simulink model "SF015A_WhlImbRejctn"  (R2013b)
settings: Solver=FixedStepDiscrete  SolverMode=SingleTasking  StartTime=0.0  StopTime=1  FixedStep=0.002  RelTol=1e-3
undefined symbols (not defined in the file): ACTIVBANDMAX_ULS_U32, ADAPVFILMAX_ULS_F32, ADJOUTPMAX_ULS_F32, ARCHGLBPRM_180OVERPI_ULS_F32, ARCHGLBPRM_2MILLISEC_SEC_F32, ARCHGLBPRM_2PI_ULS_F32, ARCHGLBPRM_FLOATZEROTHD_ULS_F32, ARCHGLBPRM_PI_ULS_F32, ARCHGLBPRM_PIOVER180_ULS_F32, ARCHGLBPRM_PIOVER2_ULS_F32, CALMINSPERCOUNT_ULS_F32, Cntr, DURATIONDISABLE_CNT_U16, FILTWHLSPDMAX_MOTRADPERSEC_F32, FRQMIN_ULS_F32, MICROSECTOMILLISEC_ULS_F32, MINSTOMILLISEC_ULS_F32, NINETY_ULS_F32, NODEBSTEP_CNT_U16, NROFDLY_CNT_U08, NtcSts1, NvmGetErrSts1, ONEHALF_ULS_F32, ONEHUNDRED_ULS_F32, ONEOVRTHREE_ULS_F32, ONEOVRTWENTY_ULS_F32, ONETHOUSAND_ULS_F32, PEAKMAX_ULS_F32, PEAKMIN_ULS_F32, PHAADJMAX_ULS_F32, PITIMESSAMPLETIME_ULS_F32, SigQlfr1, STOREDMINSPERCOUNT_ULS_F32, Sts, SysSt1, TWO_ULS_F32, TWOOVRTHREE_ULS_F32, UGRFILMAX_ULS_F32, WhlImbRejctnAdpvFac, WhlImbRejctnAutScaEna, WhlImbRejctnAutScaTar, WhlImbRejctnCurrMgnSlewPerLoop, WhlImbRejctnDcTrendFltRcvryDly, WhlImbRejctnDcTrendFltRcvryNegStep, WhlImbRejctnDcTrendFltRcvryPosStep, WhlImbRejctnDcTrendFltRcvryThd, WhlImbRejctnDcTrendTh2Tq, WhlImbRejctnDcTrendThTq, WhlImbRejctnDcTrendTi2Sec, WhlImbRejctnDcTrendTiSec, WhlImbRejctnEnaSlewPerLoop, WhlImbRejctnFctEna, WhlImbRejctnFltNtc, WhlImbRejctnFrqDiagcAmpThd, WhlImbRejctnFrqDiagcEna, WhlImbRejctnFrqDiagcFltRcvryDly, WhlImbRejctnFrqDiagcFltRcvryNegStep, WhlImbRejctnFrqDiagcFltRcvryPosStep, WhlImbRejctnFrqDiagcFltRcvryThd, WhlImbRejctnFrqDiagcThd ... (+30)
libraries: FixdToFloat x32, simulink x26, NxtrLim x25, Fil x20, NxtrAbslt x9, NxtrMath x7, NxtrMax x6, NxtrMin x4, NxtrNvM x2, FloatToFixd x2, LnrIntrpn x2, NxtrSign x1
(part 4 of 14)

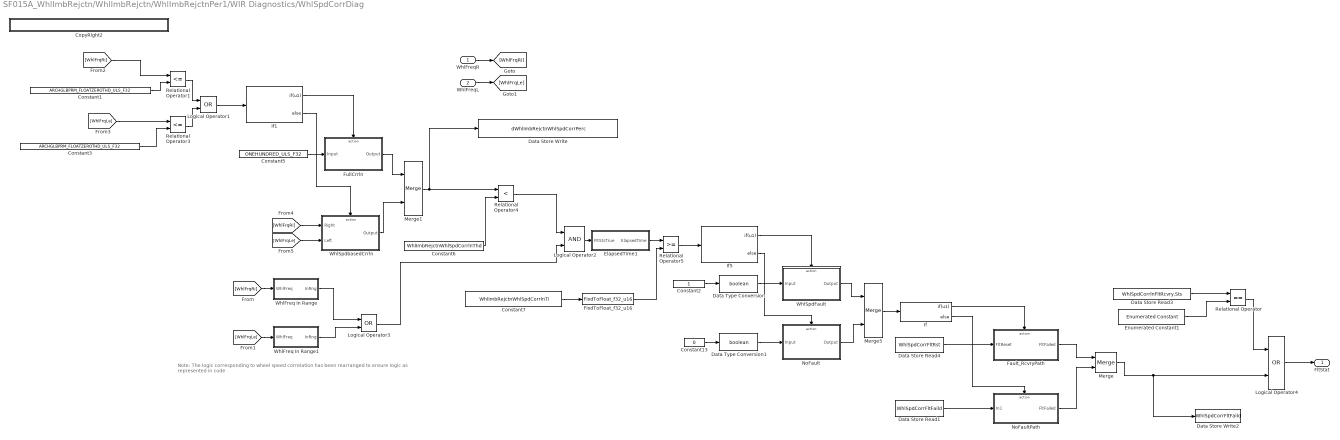
== system SF015A_WhlImbRejctn/WhlImbRejctn/WhlImbRejctnPer1/WIR Diagnostics/WhlSpdCorrDiag ==
  note: Note: The logic corresponding to wheel speed correlation has been rearranged to ensure logic as represented in code
  WhlFreqR : Inport
  WhlFreqL : Inport  Port=2
  Constant1 : Constant  Value=ARCHGLBPRM_FLOATZEROTHD_ULS_F32
  Constant13 : Constant  Value=0  OutDataTypeStr=boolean
  Constant2 : Constant  OutDataTypeStr=boolean
  Constant3 : Constant  Value=ARCHGLBPRM_FLOATZEROTHD_ULS_F32
  Constant5 : Constant  Value=ONEHUNDRED_ULS_F32
  Constant6 : Constant  Value=WhlImbRejctnWhlSpdCorrlnThd
  Constant7 : Constant  Value=WhlImbRejctnWhlSpdCorrlnTi
  CopyRight2 : Subsystem  Description=|  mask(Copyright Information){none=on}
      | Copyright info block.                                               
      |                                                                     
      | Place copyright information at the top of every subsystem in design.
      mask prompts: none "No parameters"
      mask help: Place copyright information at the top of every subsystem in design.
      mask Display:
      | NxtrConf = 'Nexteer Confidential';
      | 
      | sys = bdroot; %handle for the current model ("system")
      | first = get_param(sys,'Created');
      | first = first(end-3:end);  %year is last four digits
      | 
      | last = get_param(sys,'LastModifiedDate');
      | if isempty(last)
      |     last = datestr(now,'yyyy');
      | else
      |     last = last(end-3:end);
      | end
      | 
      | if strcmp(first,last)
      |     fprintf('%s -- Copyright %s Nexteer',NxtrConf,first)
      | else
      |     fprintf('%s -- %s%s- %s Nexteer',NxtrConf,char(169),first,last)
      | end
  Data Store Read1 : DataStoreRead  Priority=1  DataStoreName=WhlSpdCorrFltFaild
      settings: AttributesFormatString=Priority:%<Priority>
  Data Store Read3 : DataStoreRead  DataStoreName=WhlSpdCorrlnFltRcvry  DataStoreElements=WhlSpdCorrlnFltRcvry.Sts
  Data Store Read4 : DataStoreRead  Priority=1  DataStoreName=WhlSpdCorrFltRst
      settings: AttributesFormatString=Priority:%<Priority>
  Data Store Write : DataStoreWrite  DataStoreName=dWhlImbRejctnWhlSpdCorrPerc
  Data Store Write2 : DataStoreWrite  Priority=2  DataStoreName=WhlSpdCorrFltFaild
      settings: AttributesFormatString=Priority:%<Priority>
  Data Type Conversion : DataTypeConversion  OutDataTypeStr=boolean
  Data Type Conversion1 : DataTypeConversion  OutDataTypeStr=boolean
  ElapsedTime1 : Subsystem  TreatAsAtomicUnit=on
  Enumerated Constant1 : simulink/Sources/Enumerated Constant  OutDataTypeStr=Enum: SigQlfr1  Value=SigQlfr1.SIGQLFR_FAILD  SampleTime=inf
  Fault_RcvryPath : Subsystem  TreatAsAtomicUnit=on
  FixdToFloat_f32_u16 : FixdToFloat/FixdToFloat_f32_u16  Param1=0
  FullCrrln : Subsystem  RequirementInfo={} %GIDa_f316d04c_b5bf_4991_bd46_e1c3d0acec80  TreatAsAtomicUnit=on
  If : If  IfExpression=u1
  If1 : If  RequirementInfo={} %GIDa_4bc11ef0_d878_4cc4_82b4_0d0edb0129e4  IfExpression=u1
  If5 : If  RequirementInfo={} %GIDa_f8e2168d_295a_437f_93f0_d2de918d56ef  IfExpression=u1
  Logical Operator1 : Logic  Operator=OR  AllPortsSameDT=off  OutDataTypeStr=boolean
  Logical Operator2 : Logic  AllPortsSameDT=off  OutDataTypeStr=boolean
  Logical Operator3 : Logic  Operator=OR  AllPortsSameDT=off  OutDataTypeStr=boolean
  Logical Operator4 : Logic  Operator=OR  AllPortsSameDT=off  OutDataTypeStr=boolean
  Merge : Merge
  Merge1 : Merge
  Merge5 : Merge
  NoFault : Subsystem  RequirementInfo={} %GIDa_f7020847_ef3c_4257_9229_248ab4f76409  TreatAsAtomicUnit=on
  NoFaultPath : Subsystem  TreatAsAtomicUnit=on
  Relational Operator : RelationalOperator  Operator===  OutDataTypeStr=boolean
  Relational Operator1 : RelationalOperator  Operator=<=  OutDataTypeStr=boolean
  Relational Operator3 : RelationalOperator  Operator=<=  OutDataTypeStr=boolean
  Relational Operator4 : RelationalOperator  Operator=<  OutDataTypeStr=boolean
  Relational Operator5 : RelationalOperator  OutDataTypeStr=boolean
  WhlFreq In Range : Subsystem
  WhlFreq In Range1 : Subsystem
  WhlSpdFault : Subsystem  RequirementInfo={} %GIDa_32897d14_0a36_471e_bba2_f76c6f004030  TreatAsAtomicUnit=on
  WhlSpdbasedCrrln : Subsystem  RequirementInfo={} %GIDa_bfd7bd1e_da2d_43b7_9815_cea994d6f624  TreatAsAtomicUnit=on
  FltStat : Outport
  wires:
  Merge5/1 -> If/1
  Relational Operator1/1 -> Logical Operator1/1
  Relational Operator3/1 -> Logical Operator1/2
  Logical Operator1/1 -> If1/1
  Merge1/1 -> Data Store Write/1, Relational Operator4/1
  Constant6/1 -> Relational Operator4/2
  Constant7/1 -> FixdToFloat_f32_u16/1
  Relational Operator5/1 -> If5/1
  Relational Operator4/1 -> Logical Operator2/1
  WhlFreq In Range1/1(InRng) -> Logical Operator3/2
  WhlFreq In Range/1(InRng) -> Logical Operator3/1
  Logical Operator3/1 -> Logical Operator2/2
  If5/1 -> WhlSpdFault/Action
  If5/2 -> NoFault/Action
  WhlSpdFault/1(Output) -> Merge5/1
  NoFault/1(Output) -> Merge5/2
  Constant2/1 -> Data Type Conversion/1
  Constant13/1 -> Data Type Conversion1/1
  If1/1 -> FullCrrln/Action
  If1/2 -> WhlSpdbasedCrrln/Action
  FullCrrln/1(Output) -> Merge1/1
  WhlSpdbasedCrrln/1(Output) -> Merge1/2
  Constant5/1 -> FullCrrln/1(Input)
  ElapsedTime1/1(ElapsedTime) -> Relational Operator5/1
  Logical Operator2/1 -> ElapsedTime1/1(FltStsTrue)
  FixdToFloat_f32_u16/1 -> Relational Operator5/2
  Data Type Conversion/1 -> WhlSpdFault/1(Input)
  Data Type Conversion1/1 -> NoFault/1(Input)
  Constant3/1 -> Relational Operator3/2
  Constant1/1 -> Relational Operator1/2
  WhlFreqR/1 -> [WhlFrqRi]
  WhlFreqL/1 -> [WhlFrqLe]
  [WhlFrqRi] -> WhlFreq In Range/1(WhlFreq)
  [WhlFrqLe] -> WhlFreq In Range1/1(WhlFreq)
  [WhlFrqLe] -> Relational Operator3/1
  [WhlFrqRi] -> Relational Operator1/1
  [WhlFrqLe] -> WhlSpdbasedCrrln/2(Left)
  [WhlFrqRi] -> WhlSpdbasedCrrln/1(Right)
  Data Store Read4/1 -> Fault_RcvryPath/1(FltReset)
  If/1 -> Fault_RcvryPath/Action
  Fault_RcvryPath/1(FltFailed) -> Merge/1
  NoFaultPath/1(FltFailed) -> Merge/2
  If/2 -> NoFaultPath/Action
  Enumerated Constant1/1 -> Relational Operator/2
  Relational Operator/1 -> Logical Operator4/1
  Data Store Read3/1 -> Relational Operator/1
  Logical Operator4/1 -> FltStat/1
  Merge/1 -> Data Store Write2/1, Logical Operator4/2
  Data Store Read1/1 -> NoFaultPath/1(In1)

== system SF015A_WhlImbRejctn/WhlImbRejctn/WhlImbRejctnPer1/Whl Spd filter and Freq Estimation/CopyRight2 ==

== system SF015A_WhlImbRejctn/WhlImbRejctn/WhlImbRejctnPer1/Whl Spd filter and Freq Estimation/Tapped Delay ImplementationLe ==
  Input : Inport
  30 Delay's Execution : Subsystem  Priority=1  TreatAsAtomicUnit=on
      settings: AttributesFormatString=Priority:%<Priority>
  Assignment1 : Assignment  IndexMode=Zero-based  IndexOptions=Index vector (port)  Indices=1  OutputSizes=1
  Constant1 : Constant  Value=NROFDLY_CNT_U08  OutDataTypeStr=uint8
      settings: AttributesFormatString=%<OutDataTypeStr>
  CopyRight2 : Subsystem  Description=|  mask(Copyright Information){none=on}
      | Copyright info block.                                               
      |                                                                     
      | Place copyright information at the top of every subsystem in design.
      mask prompts: none "No parameters"
      mask help: Place copyright information at the top of every subsystem in design.
      mask Display:
      | NxtrConf = 'Nexteer Confidential';
      | 
      | sys = bdroot; %handle for the current model ("system")
      | first = get_param(sys,'Created');
      | first = first(end-3:end);  %year is last four digits
      | 
      | last = get_param(sys,'LastModifiedDate');
      | if isempty(last)
      |     last = datestr(now,'yyyy');
      | else
      |     last = last(end-3:end);
      | end
      | 
      | if strcmp(first,last)
      |     fprintf('%s -- Copyright %s Nexteer',NxtrConf,first)
      | else
      |     fprintf('%s -- %s%s- %s Nexteer',NxtrConf,char(169),first,last)
      | end
  Data Store Read1 : DataStoreRead  Priority=4  DataStoreName=StordValLe
      settings: AttributesFormatString=Priority=%<Priority>
  Data Store Read3 : DataStoreRead  Priority=2  DataStoreName=StordValLe
      settings: AttributesFormatString=Priority=%<Priority>
  Data Store Write : DataStoreWrite  Priority=3  DataStoreName=StordValLe
      settings: AttributesFormatString=Priority=%<Priority>
  Tapped Signal : Outport
  wires:
  Input/1 -> Assignment1/2
  Constant1/1 -> Assignment1/3
  Data Store Read3/1 -> Assignment1/1
  Assignment1/1 -> Data Store Write/1
  Data Store Read1/1 -> Tapped Signal/1

== system SF015A_WhlImbRejctn/WhlImbRejctn/WhlImbRejctnPer1/Whl Spd filter and Freq Estimation/Tapped Delay ImplementationRi ==
  Input : Inport
  30 Delay's Execution : Subsystem  Priority=1  TreatAsAtomicUnit=on
      settings: AttributesFormatString=Priority:%<Priority>
  Assignment1 : Assignment  IndexMode=Zero-based  IndexOptions=Index vector (port)  Indices=1  OutputSizes=1
  Constant1 : Constant  Value=NROFDLY_CNT_U08  OutDataTypeStr=uint8
      settings: AttributesFormatString=%<OutDataTypeStr>
  CopyRight2 : Subsystem  Description=|  mask(Copyright Information){none=on}
      | Copyright info block.                                               
      |                                                                     
      | Place copyright information at the top of every subsystem in design.
      mask prompts: none "No parameters"
      mask help: Place copyright information at the top of every subsystem in design.
      mask Display:
      | NxtrConf = 'Nexteer Confidential';
      | 
      | sys = bdroot; %handle for the current model ("system")
      | first = get_param(sys,'Created');
      | first = first(end-3:end);  %year is last four digits
      | 
      | last = get_param(sys,'LastModifiedDate');
      | if isempty(last)
      |     last = datestr(now,'yyyy');
      | else
      |     last = last(end-3:end);
      | end
      | 
      | if strcmp(first,last)
      |     fprintf('%s -- Copyright %s Nexteer',NxtrConf,first)
      | else
      |     fprintf('%s -- %s%s- %s Nexteer',NxtrConf,char(169),first,last)
      | end
  Data Store Read1 : DataStoreRead  Priority=4  DataStoreName=StordValRi
      settings: AttributesFormatString=Priority=%<Priority>
  Data Store Read3 : DataStoreRead  Priority=2  DataStoreName=StordValRi
      settings: AttributesFormatString=Priority=%<Priority>
  Data Store Write : DataStoreWrite  Priority=3  DataStoreName=StordValRi
      settings: AttributesFormatString=Priority=%<Priority>
  Tapped Signal : Outport
  wires:
  Input/1 -> Assignment1/2
  Constant1/1 -> Assignment1/3
  Data Store Read3/1 -> Assignment1/1
  Assignment1/1 -> Data Store Write/1
  Data Store Read1/1 -> Tapped Signal/1

== system SF015A_WhlImbRejctn/WhlImbRejctn/WhlImbRejctnPer1/Whl Spd filter and Freq Estimation/UGR L ==
  y : Inport
  FreqEst_Hz : Inport  Port=2
  PoleMag : Inport  Port=3
  Calc_ma1_a2 : Subsystem
  CopyRight2 : Subsystem  Description=|  mask(Copyright Information){none=on}
      | Copyright info block.                                               
      |                                                                     
      | Place copyright information at the top of every subsystem in design.
      mask prompts: none "No parameters"
      mask help: Place copyright information at the top of every subsystem in design.
      mask Display:
      | NxtrConf = 'Nexteer Confidential';
      | 
      | sys = bdroot; %handle for the current model ("system")
      | first = get_param(sys,'Created');
      | first = first(end-3:end);  %year is last four digits
      | 
      | last = get_param(sys,'LastModifiedDate');
      | if isempty(last)
      |     last = datestr(now,'yyyy');
      | else
      |     last = last(end-3:end);
      | end
      | 
      | if strcmp(first,last)
      |     fprintf('%s -- Copyright %s Nexteer',NxtrConf,first)
      | else
      |     fprintf('%s -- %s%s- %s Nexteer',NxtrConf,char(169),first,last)
      | end
  UnityGainResFilt : Subsystem
  y Filt : Outport
  wires:
  y/1 -> UnityGainResFilt/1(y)
  FreqEst_Hz/1 -> Calc_ma1_a2/1(f_est)
  UnityGainResFilt/1(Filt) -> y Filt/1
  Calc_ma1_a2/1(minus_a1) -> UnityGainResFilt/2(minus_a1)
  Calc_ma1_a2/2(a2) -> UnityGainResFilt/3(a2)
  PoleMag/1 -> Calc_ma1_a2/2(PoleMag)

== system SF015A_WhlImbRejctn/WhlImbRejctn/WhlImbRejctnPer1/Whl Spd filter and Freq Estimation/UGR R ==
  y : Inport
  FreqEst_Hz : Inport  Port=2
  PoleMag : Inport  Port=3
  Calc_ma1_a2 : Subsystem
  CopyRight2 : Subsystem  Description=|  mask(Copyright Information){none=on}
      | Copyright info block.                                               
      |                                                                     
      | Place copyright information at the top of every subsystem in design.
      mask prompts: none "No parameters"
      mask help: Place copyright information at the top of every subsystem in design.
      mask Display:
      | NxtrConf = 'Nexteer Confidential';
      | 
      | sys = bdroot; %handle for the current model ("system")
      | first = get_param(sys,'Created');
      | first = first(end-3:end);  %year is last four digits
      | 
      | last = get_param(sys,'LastModifiedDate');
      | if isempty(last)
      |     last = datestr(now,'yyyy');
      | else
      |     last = last(end-3:end);
      | end
      | 
      | if strcmp(first,last)
      |     fprintf('%s -- Copyright %s Nexteer',NxtrConf,first)
      | else
      |     fprintf('%s -- %s%s- %s Nexteer',NxtrConf,char(169),first,last)
      | end
  UnityGainResFilt : Subsystem
  y Filt : Outport
  wires:
  y/1 -> UnityGainResFilt/1(y)
  FreqEst_Hz/1 -> Calc_ma1_a2/1(f_est)
  UnityGainResFilt/1(Filt) -> y Filt/1
  Calc_ma1_a2/1(minus_a1) -> UnityGainResFilt/2(minus_a1)
  Calc_ma1_a2/2(a2) -> UnityGainResFilt/3(a2)
  PoleMag/1 -> Calc_ma1_a2/2(PoleMag)

== system SF015A_WhlImbRejctn/WhlImbRejctn/WhlImbRejctnPer2/Flt Recovery- DC Trend/CopyRight2 ==

== system SF015A_WhlImbRejctn/WhlImbRejctn/WhlImbRejctnPer2/Flt Recovery- DC Trend/ElapsedTime1 ==
  FltStsTrue : Inport
  CopyRight2 : Subsystem  Description=|  mask(Copyright Information){none=on}
      | Copyright info block.                                               
      |                                                                     
      | Place copyright information at the top of every subsystem in design.
      mask prompts: none "No parameters"
      mask help: Place copyright information at the top of every subsystem in design.
      mask Display:
      | NxtrConf = 'Nexteer Confidential';
      | 
      | sys = bdroot; %handle for the current model ("system")
      | first = get_param(sys,'Created');
      | first = first(end-3:end);  %year is last four digits
      | 
      | last = get_param(sys,'LastModifiedDate');
      | if isempty(last)
      |     last = datestr(now,'yyyy');
      | else
      |     last = last(end-3:end);
      | end
      | 
      | if strcmp(first,last)
      |     fprintf('%s -- Copyright %s Nexteer',NxtrConf,first)
      | else
      |     fprintf('%s -- %s%s- %s Nexteer',NxtrConf,char(169),first,last)
      | end
  Data Store Read : DataStoreRead  Priority=1  DataStoreName=DcTrendLrngEnaPrev
      settings: AttributesFormatString="priority:  %<Priority>"
  Data Store Write : DataStoreWrite  Priority=2  DataStoreName=DcTrendLrngEnaPrev
      settings: AttributesFormatString="priority:  %<Priority>"
  If : If  NumInputs=2  IfExpression=u1  ElseIfExpressions=u2
  If not true elapsed time = 0 : Subsystem  TreatAsAtomicUnit=on
  "If true and last step is true calculate elapsed time " : Subsystem  TreatAsAtomicUnit=on
  "If true and last step not true elapsed time = 0 get reference time " : Subsystem  TreatAsAtomicUnit=on
  Logical Operator1 : Logic  Operator=NOT  AllPortsSameDT=off  OutDataTypeStr=boolean
  Logical Operator2 : Logic  Operator=NOT  AllPortsSameDT=off  OutDataTypeStr=boolean
  Merge : Merge  Inputs=3
  ElapsedTime : Outport
  wires:
  If/1 -> If not true elapsed time = 0/Action
  If/2 -> "If true and last step not true elapsed time = 0 get reference time "/Action
  If/3 -> "If true and last step is true calculate elapsed time "/Action
  If not true elapsed time = 0/1(SpanTi) -> Merge/1
  "If true and last step not true elapsed time = 0 get reference time "/1("SpanTi ") -> Merge/2
  "If true and last step is true calculate elapsed time "/1(SpanTi) -> Merge/3
  Merge/1 -> ElapsedTime/1
  FltStsTrue/1 -> Logical Operator2/1, Data Store Write/1
  Data Store Read/1 -> Logical Operator1/1
  Logical Operator2/1 -> If/1
  Logical Operator1/1 -> If/2

== system SF015A_WhlImbRejctn/WhlImbRejctn/WhlImbRejctnPer2/Flt Recovery- DC Trend/FaultReset_Rcvry_False ==
  Action Port : ActionPort  ActionType=else
  Constant1 : Constant  Value=0  OutDataTypeStr=boolean
  CopyRight2 : Subsystem  Description=|  mask(Copyright Information){none=on}
      | Copyright info block.                                               
      |                                                                     
      | Place copyright information at the top of every subsystem in design.
      mask prompts: none "No parameters"
      mask help: Place copyright information at the top of every subsystem in design.
      mask Display:
      | NxtrConf = 'Nexteer Confidential';
      | 
      | sys = bdroot; %handle for the current model ("system")
      | first = get_param(sys,'Created');
      | first = first(end-3:end);  %year is last four digits
      | 
      | last = get_param(sys,'LastModifiedDate');
      | if isempty(last)
      |     last = datestr(now,'yyyy');
      | else
      |     last = last(end-3:end);
      | end
      | 
      | if strcmp(first,last)
      |     fprintf('%s -- Copyright %s Nexteer',NxtrConf,first)
      | else
      |     fprintf('%s -- %s%s- %s Nexteer',NxtrConf,char(169),first,last)
      | end
  Out1 : Outport
  wires:
  Constant1/1 -> Out1/1

== system SF015A_WhlImbRejctn/WhlImbRejctn/WhlImbRejctnPer2/Flt Recovery- DC Trend/FaultReset_Rcvry_True ==
  Action Port : ActionPort  ActionType=then
  Constant15 : Constant  OutDataTypeStr=boolean
  CopyRight2 : Subsystem  Description=|  mask(Copyright Information){none=on}
      | Copyright info block.                                               
      |                                                                     
      | Place copyright information at the top of every subsystem in design.
      mask prompts: none "No parameters"
      mask help: Place copyright information at the top of every subsystem in design.
      mask Display:
      | NxtrConf = 'Nexteer Confidential';
      | 
      | sys = bdroot; %handle for the current model ("system")
      | first = get_param(sys,'Created');
      | first = first(end-3:end);  %year is last four digits
      | 
      | last = get_param(sys,'LastModifiedDate');
      | if isempty(last)
      |     last = datestr(now,'yyyy');
      | else
      |     last = last(end-3:end);
      | end
      | 
      | if strcmp(first,last)
      |     fprintf('%s -- Copyright %s Nexteer',NxtrConf,first)
      | else
      |     fprintf('%s -- %s%s- %s Nexteer',NxtrConf,char(169),first,last)
      | end
  Out1 : Outport
  wires:
  Constant15/1 -> Out1/1

== system SF015A_WhlImbRejctn/WhlImbRejctn/WhlImbRejctnPer2/Flt Recovery- DC Trend/Update Fault Status ==
  Structvar : Inport
  Status : Inport  Port=2
  Bus Assignment : BusAssignment  AssignedSignals=Cntr,Sts
  Bus Selector : BusSelector  OutputSignals=Cntr,Sts,Thd,NegStep,PosStep
  Compare To Zero : simulink/Logic and Bit Operations/Compare To Zero  relop=<=  OutDataTypeStr=boolean
  Constant : Constant  Value=0  OutDataTypeStr=single
  CopyRight2 : Subsystem  Description=|  mask(Copyright Information){none=on}
      | Copyright info block.                                               
      |                                                                     
      | Place copyright information at the top of every subsystem in design.
      mask prompts: none "No parameters"
      mask help: Place copyright information at the top of every subsystem in design.
      mask Display:
      | NxtrConf = 'Nexteer Confidential';
      | 
      | sys = bdroot; %handle for the current model ("system")
      | first = get_param(sys,'Created');
      | first = first(end-3:end);  %year is last four digits
      | 
      | last = get_param(sys,'LastModifiedDate');
      | if isempty(last)
      |     last = datestr(now,'yyyy');
      | else
      |     last = last(end-3:end);
      | end
      | 
      | if strcmp(first,last)
      |     fprintf('%s -- Copyright %s Nexteer',NxtrConf,first)
      | else
      |     fprintf('%s -- %s%s- %s Nexteer',NxtrConf,char(169),first,last)
      | end
  Enumerated Constant : simulink/Sources/Enumerated Constant  OutDataTypeStr=Enum: SigQlfr1  Value=SigQlfr1.SIGQLFR_FAILD  SampleTime=inf
  Enumerated Constant1 : simulink/Sources/Enumerated Constant  OutDataTypeStr=Enum: SigQlfr1  Value=SigQlfr1.SIGQLFR_PASSD  SampleTime=inf
  If : If  IfExpression=u1
  If1 : If  NumInputs=2  IfExpression=u1  ElseIfExpressions=u2  ShowElse=off
  Merge : Merge
  Relational Operator : RelationalOperator  OutDataTypeStr=boolean
  Terminator : Terminator
  Towards Failed : Subsystem  TreatAsAtomicUnit=on
  Towards Passed : Subsystem  TreatAsAtomicUnit=on
  Update to Failed : Subsystem  TreatAsAtomicUnit=on
  Update to Passed : Subsystem  TreatAsAtomicUnit=on
  counter : Merge
  Structvar_out : Outport
  wires:
  Structvar/1 -> Bus Assignment/1, Bus Selector/1
  Status/1 -> If/1
  If/1 -> Towards Failed/Action
  If/2 -> Towards Passed/Action
  [PosStep] -> Towards Failed/1(PosStep)
  [NegStep] -> Towards Passed/1(NegStep)
  Towards Failed/1(Out1) -> counter/1
  Towards Passed/1(Out1) -> counter/2
  [Cnt] -> Towards Failed/2(Cnt)
  [Thd] -> Towards Failed/3(Thd)
  Constant/1 -> Towards Passed/3(Thd)
  counter/1 -> [Cnt_update], Compare To Zero/1, Relational Operator/1
  Relational Operator/1 -> If1/1
  If1/1 -> Update to Failed/Action
  If1/2 -> Update to Passed/Action
  Compare To Zero/1 -> If1/2
  Enumerated Constant1/1 -> Update to Passed/1(In1)
  Update to Failed/1(Out1) -> Merge/1
  Update to Passed/1(Out1) -> Merge/2
  Enumerated Constant/1 -> Update to Failed/1(In1)
  Bus Assignment/1 -> Structvar_out/1
  Merge/1 -> [Sts_update]
  Bus Selector/1 -> [Cnt]  "<Cntr>"
  Bus Selector/3 -> [Thd]  "<Thd>"
  Bus Selector/4 -> [NegStep]  "<NegStep>"
  Bus Selector/5 -> [PosStep]  "<PosStep>"
  [Cnt_update] -> Bus Assignment/2
  [Sts_update] -> Bus Assignment/3
  [Cnt] -> Towards Passed/2(Cnt)
  [Thd] -> Relational Operator/2
  Bus Selector/2 -> Terminator/1  "<Sts>"

== system SF015A_WhlImbRejctn/WhlImbRejctn/WhlImbRejctnPer2/Flt Recovery- Freq Diag/CopyRight2 ==

== system SF015A_WhlImbRejctn/WhlImbRejctn/WhlImbRejctnPer2/Flt Recovery- Freq Diag/ElapsedTime1 ==
  FltStsTrue : Inport
  CopyRight2 : Subsystem  Description=|  mask(Copyright Information){none=on}
      | Copyright info block.                                               
      |                                                                     
      | Place copyright information at the top of every subsystem in design.
      mask prompts: none "No parameters"
      mask help: Place copyright information at the top of every subsystem in design.
      mask Display:
      | NxtrConf = 'Nexteer Confidential';
      | 
      | sys = bdroot; %handle for the current model ("system")
      | first = get_param(sys,'Created');
      | first = first(end-3:end);  %year is last four digits
      | 
      | last = get_param(sys,'LastModifiedDate');
      | if isempty(last)
      |     last = datestr(now,'yyyy');
      | else
      |     last = last(end-3:end);
      | end
      | 
      | if strcmp(first,last)
      |     fprintf('%s -- Copyright %s Nexteer',NxtrConf,first)
      | else
      |     fprintf('%s -- %s%s- %s Nexteer',NxtrConf,char(169),first,last)
      | end
  Data Store Read : DataStoreRead  Priority=1  DataStoreName=FrqDiagcLrngEnaPrev
      settings: AttributesFormatString="priority:  %<Priority>"
  Data Store Write : DataStoreWrite  Priority=2  DataStoreName=FrqDiagcLrngEnaPrev
      settings: AttributesFormatString="priority:  %<Priority>"
  If : If  NumInputs=2  IfExpression=u1  ElseIfExpressions=u2
  If not true elapsed time = 0 : Subsystem  TreatAsAtomicUnit=on
  "If true and last step is true calculate elapsed time " : Subsystem  TreatAsAtomicUnit=on
  "If true and last step not true elapsed time = 0 get reference time " : Subsystem  TreatAsAtomicUnit=on
  Logical Operator1 : Logic  Operator=NOT  AllPortsSameDT=off  OutDataTypeStr=boolean
  Logical Operator2 : Logic  Operator=NOT  AllPortsSameDT=off  OutDataTypeStr=boolean
  Merge : Merge  Inputs=3
  ElapsedTime : Outport
  wires:
  If/1 -> If not true elapsed time = 0/Action
  If/2 -> "If true and last step not true elapsed time = 0 get reference time "/Action
  If/3 -> "If true and last step is true calculate elapsed time "/Action
  If not true elapsed time = 0/1(SpanTi) -> Merge/1
  "If true and last step not true elapsed time = 0 get reference time "/1("SpanTi ") -> Merge/2
  "If true and last step is true calculate elapsed time "/1(SpanTi) -> Merge/3
  Merge/1 -> ElapsedTime/1
  FltStsTrue/1 -> Logical Operator2/1, Data Store Write/1
  Data Store Read/1 -> Logical Operator1/1
  Logical Operator2/1 -> If/1
  Logical Operator1/1 -> If/2

== system SF015A_WhlImbRejctn/WhlImbRejctn/WhlImbRejctnPer2/Flt Recovery- Freq Diag/FaultReset_Rcvry_False ==
  Action Port : ActionPort  ActionType=else
  Constant1 : Constant  Value=0  OutDataTypeStr=boolean
  CopyRight2 : Subsystem  Description=|  mask(Copyright Information){none=on}
      | Copyright info block.                                               
      |                                                                     
      | Place copyright information at the top of every subsystem in design.
      mask prompts: none "No parameters"
      mask help: Place copyright information at the top of every subsystem in design.
      mask Display:
      | NxtrConf = 'Nexteer Confidential';
      | 
      | sys = bdroot; %handle for the current model ("system")
      | first = get_param(sys,'Created');
      | first = first(end-3:end);  %year is last four digits
      | 
      | last = get_param(sys,'LastModifiedDate');
      | if isempty(last)
      |     last = datestr(now,'yyyy');
      | else
      |     last = last(end-3:end);
      | end
      | 
      | if strcmp(first,last)
      |     fprintf('%s -- Copyright %s Nexteer',NxtrConf,first)
      | else
      |     fprintf('%s -- %s%s- %s Nexteer',NxtrConf,char(169),first,last)
      | end
  Out1 : Outport
  wires:
  Constant1/1 -> Out1/1

== system SF015A_WhlImbRejctn/WhlImbRejctn/WhlImbRejctnPer2/Flt Recovery- Freq Diag/FaultReset_Rcvry_True ==
  Action Port : ActionPort  ActionType=then
  Constant15 : Constant  OutDataTypeStr=boolean
  CopyRight2 : Subsystem  Description=|  mask(Copyright Information){none=on}
      | Copyright info block.                                               
      |                                                                     
      | Place copyright information at the top of every subsystem in design.
      mask prompts: none "No parameters"
      mask help: Place copyright information at the top of every subsystem in design.
      mask Display:
      | NxtrConf = 'Nexteer Confidential';
      | 
      | sys = bdroot; %handle for the current model ("system")
      | first = get_param(sys,'Created');
      | first = first(end-3:end);  %year is last four digits
      | 
      | last = get_param(sys,'LastModifiedDate');
      | if isempty(last)
      |     last = datestr(now,'yyyy');
      | else
      |     last = last(end-3:end);
      | end
      | 
      | if strcmp(first,last)
      |     fprintf('%s -- Copyright %s Nexteer',NxtrConf,first)
      | else
      |     fprintf('%s -- %s%s- %s Nexteer',NxtrConf,char(169),first,last)
      | end
  Out1 : Outport
  wires:
  Constant15/1 -> Out1/1

== system SF015A_WhlImbRejctn/WhlImbRejctn/WhlImbRejctnPer2/Flt Recovery- Freq Diag/Update Fault Status ==
  Structvar : Inport
  Status : Inport  Port=2
  Bus Assignment : BusAssignment  AssignedSignals=Cntr,Sts
  Bus Selector : BusSelector  OutputSignals=Cntr,Sts,Thd,NegStep,PosStep
  Compare To Zero : simulink/Logic and Bit Operations/Compare To Zero  relop=<=  OutDataTypeStr=boolean
  Constant : Constant  Value=0  OutDataTypeStr=single
  CopyRight2 : Subsystem  Description=|  mask(Copyright Information){none=on}
      | Copyright info block.                                               
      |                                                                     
      | Place copyright information at the top of every subsystem in design.
      mask prompts: none "No parameters"
      mask help: Place copyright information at the top of every subsystem in design.
      mask Display:
      | NxtrConf = 'Nexteer Confidential';
      | 
      | sys = bdroot; %handle for the current model ("system")
      | first = get_param(sys,'Created');
      | first = first(end-3:end);  %year is last four digits
      | 
      | last = get_param(sys,'LastModifiedDate');
      | if isempty(last)
      |     last = datestr(now,'yyyy');
      | else
      |     last = last(end-3:end);
      | end
      | 
      | if strcmp(first,last)
      |     fprintf('%s -- Copyright %s Nexteer',NxtrConf,first)
      | else
      |     fprintf('%s -- %s%s- %s Nexteer',NxtrConf,char(169),first,last)
      | end
  Enumerated Constant : simulink/Sources/Enumerated Constant  OutDataTypeStr=Enum: SigQlfr1  Value=SigQlfr1.SIGQLFR_FAILD  SampleTime=inf
  Enumerated Constant1 : simulink/Sources/Enumerated Constant  OutDataTypeStr=Enum: SigQlfr1  Value=SigQlfr1.SIGQLFR_PASSD  SampleTime=inf
  If : If  IfExpression=u1
  If1 : If  NumInputs=2  IfExpression=u1  ElseIfExpressions=u2  ShowElse=off
  Merge : Merge
  Relational Operator : RelationalOperator  OutDataTypeStr=boolean
  Terminator : Terminator
  Towards Failed : Subsystem  TreatAsAtomicUnit=on
  Towards Passed : Subsystem  TreatAsAtomicUnit=on
  Update to Failed : Subsystem  TreatAsAtomicUnit=on
  Update to Passed : Subsystem  TreatAsAtomicUnit=on
  counter : Merge
  Structvar_out : Outport
  wires:
  Structvar/1 -> Bus Assignment/1, Bus Selector/1
  Status/1 -> If/1
  If/1 -> Towards Failed/Action
  If/2 -> Towards Passed/Action
  [PosStep] -> Towards Failed/1(PosStep)
  [NegStep] -> Towards Passed/1(NegStep)
  Towards Failed/1(Out1) -> counter/1
  Towards Passed/1(Out1) -> counter/2
  [Cnt] -> Towards Failed/2(Cnt)
  [Thd] -> Towards Failed/3(Thd)
  Constant/1 -> Towards Passed/3(Thd)
  counter/1 -> [Cnt_update], Compare To Zero/1, Relational Operator/1
  Relational Operator/1 -> If1/1
  If1/1 -> Update to Failed/Action
  If1/2 -> Update to Passed/Action
  Compare To Zero/1 -> If1/2
  Enumerated Constant1/1 -> Update to Passed/1(In1)
  Update to Failed/1(Out1) -> Merge/1
  Update to Passed/1(Out1) -> Merge/2
  Enumerated Constant/1 -> Update to Failed/1(In1)
  Bus Assignment/1 -> Structvar_out/1
  Merge/1 -> [Sts_update]
  Bus Selector/1 -> [Cnt]  "<Cntr>"
  Bus Selector/3 -> [Thd]  "<Thd>"
  Bus Selector/4 -> [NegStep]  "<NegStep>"
  Bus Selector/5 -> [PosStep]  "<PosStep>"
  [Cnt_update] -> Bus Assignment/2
  [Sts_update] -> Bus Assignment/3
  [Cnt] -> Towards Passed/2(Cnt)
  [Thd] -> Relational Operator/2
  Bus Selector/2 -> Terminator/1  "<Sts>"

== system SF015A_WhlImbRejctn/WhlImbRejctn/WhlImbRejctnPer2/Flt Recovery- Max Mag/CopyRight2 ==

== system SF015A_WhlImbRejctn/WhlImbRejctn/WhlImbRejctnPer2/Flt Recovery- Max Mag/ElapsedTime1 ==
  FltStsTrue : Inport
  CopyRight2 : Subsystem  Description=|  mask(Copyright Information){none=on}
      | Copyright info block.                                               
      |                                                                     
      | Place copyright information at the top of every subsystem in design.
      mask prompts: none "No parameters"
      mask help: Place copyright information at the top of every subsystem in design.
      mask Display:
      | NxtrConf = 'Nexteer Confidential';
      | 
      | sys = bdroot; %handle for the current model ("system")
      | first = get_param(sys,'Created');
      | first = first(end-3:end);  %year is last four digits
      | 
      | last = get_param(sys,'LastModifiedDate');
      | if isempty(last)
      |     last = datestr(now,'yyyy');
      | else
      |     last = last(end-3:end);
      | end
      | 
      | if strcmp(first,last)
      |     fprintf('%s -- Copyright %s Nexteer',NxtrConf,first)
      | else
      |     fprintf('%s -- %s%s- %s Nexteer',NxtrConf,char(169),first,last)
      | end
  Data Store Read : DataStoreRead  Priority=1  DataStoreName=MaxMgnLrngEnaPrev
      settings: AttributesFormatString="priority:  %<Priority>"
  Data Store Write : DataStoreWrite  Priority=2  DataStoreName=MaxMgnLrngEnaPrev
      settings: AttributesFormatString="priority:  %<Priority>"
  If : If  NumInputs=2  IfExpression=u1  ElseIfExpressions=u2
  If not true elapsed time = 0 : Subsystem  TreatAsAtomicUnit=on
  "If true and last step is true calculate elapsed time " : Subsystem  TreatAsAtomicUnit=on
  "If true and last step not true elapsed time = 0 get reference time " : Subsystem  TreatAsAtomicUnit=on
  Logical Operator1 : Logic  Operator=NOT  AllPortsSameDT=off  OutDataTypeStr=boolean
  Logical Operator2 : Logic  Operator=NOT  AllPortsSameDT=off  OutDataTypeStr=boolean
  Merge : Merge  Inputs=3
  ElapsedTime : Outport
  wires:
  If/1 -> If not true elapsed time = 0/Action
  If/2 -> "If true and last step not true elapsed time = 0 get reference time "/Action
  If/3 -> "If true and last step is true calculate elapsed time "/Action
  If not true elapsed time = 0/1(SpanTi) -> Merge/1
  "If true and last step not true elapsed time = 0 get reference time "/1("SpanTi ") -> Merge/2
  "If true and last step is true calculate elapsed time "/1(SpanTi) -> Merge/3
  Merge/1 -> ElapsedTime/1
  FltStsTrue/1 -> Logical Operator2/1, Data Store Write/1
  Data Store Read/1 -> Logical Operator1/1
  Logical Operator2/1 -> If/1
  Logical Operator1/1 -> If/2

== system SF015A_WhlImbRejctn/WhlImbRejctn/WhlImbRejctnPer2/Flt Recovery- Max Mag/FaultReset_Rcvry_False ==
  Action Port : ActionPort  ActionType=else
  Constant1 : Constant  Value=0  OutDataTypeStr=boolean
  CopyRight2 : Subsystem  Description=|  mask(Copyright Information){none=on}
      | Copyright info block.                                               
      |                                                                     
      | Place copyright information at the top of every subsystem in design.
      mask prompts: none "No parameters"
      mask help: Place copyright information at the top of every subsystem in design.
      mask Display:
      | NxtrConf = 'Nexteer Confidential';
      | 
      | sys = bdroot; %handle for the current model ("system")
      | first = get_param(sys,'Created');
      | first = first(end-3:end);  %year is last four digits
      | 
      | last = get_param(sys,'LastModifiedDate');
      | if isempty(last)
      |     last = datestr(now,'yyyy');
      | else
      |     last = last(end-3:end);
      | end
      | 
      | if strcmp(first,last)
      |     fprintf('%s -- Copyright %s Nexteer',NxtrConf,first)
      | else
      |     fprintf('%s -- %s%s- %s Nexteer',NxtrConf,char(169),first,last)
      | end
  Out1 : Outport
  wires:
  Constant1/1 -> Out1/1

== system SF015A_WhlImbRejctn/WhlImbRejctn/WhlImbRejctnPer2/Flt Recovery- Max Mag/FaultReset_Rcvry_True ==
  Action Port : ActionPort  ActionType=then
  Constant15 : Constant  OutDataTypeStr=boolean
  CopyRight2 : Subsystem  Description=|  mask(Copyright Information){none=on}
      | Copyright info block.                                               
      |                                                                     
      | Place copyright information at the top of every subsystem in design.
      mask prompts: none "No parameters"
      mask help: Place copyright information at the top of every subsystem in design.
      mask Display:
      | NxtrConf = 'Nexteer Confidential';
      | 
      | sys = bdroot; %handle for the current model ("system")
      | first = get_param(sys,'Created');
      | first = first(end-3:end);  %year is last four digits
      | 
      | last = get_param(sys,'LastModifiedDate');
      | if isempty(last)
      |     last = datestr(now,'yyyy');
      | else
      |     last = last(end-3:end);
      | end
      | 
      | if strcmp(first,last)
      |     fprintf('%s -- Copyright %s Nexteer',NxtrConf,first)
      | else
      |     fprintf('%s -- %s%s- %s Nexteer',NxtrConf,char(169),first,last)
      | end
  Out1 : Outport
  wires:
  Constant15/1 -> Out1/1

== system SF015A_WhlImbRejctn/WhlImbRejctn/WhlImbRejctnPer2/Flt Recovery- Max Mag/Update Fault Status ==
  Structvar : Inport
  Status : Inport  Port=2
  Bus Assignment : BusAssignment  AssignedSignals=Cntr,Sts
  Bus Selector : BusSelector  OutputSignals=Cntr,Sts,Thd,NegStep,PosStep
  Compare To Zero : simulink/Logic and Bit Operations/Compare To Zero  relop=<=  OutDataTypeStr=boolean
  Constant : Constant  Value=0  OutDataTypeStr=single
  CopyRight2 : Subsystem  Description=|  mask(Copyright Information){none=on}
      | Copyright info block.                                               
      |                                                                     
      | Place copyright information at the top of every subsystem in design.
      mask prompts: none "No parameters"
      mask help: Place copyright information at the top of every subsystem in design.
      mask Display:
      | NxtrConf = 'Nexteer Confidential';
      | 
      | sys = bdroot; %handle for the current model ("system")
      | first = get_param(sys,'Created');
      | first = first(end-3:end);  %year is last four digits
      | 
      | last = get_param(sys,'LastModifiedDate');
      | if isempty(last)
      |     last = datestr(now,'yyyy');
      | else
      |     last = last(end-3:end);
      | end
      | 
      | if strcmp(first,last)
      |     fprintf('%s -- Copyright %s Nexteer',NxtrConf,first)
      | else
      |     fprintf('%s -- %s%s- %s Nexteer',NxtrConf,char(169),first,last)
      | end
  Enumerated Constant : simulink/Sources/Enumerated Constant  OutDataTypeStr=Enum: SigQlfr1  Value=SigQlfr1.SIGQLFR_FAILD  SampleTime=inf
  Enumerated Constant1 : simulink/Sources/Enumerated Constant  OutDataTypeStr=Enum: SigQlfr1  Value=SigQlfr1.SIGQLFR_PASSD  SampleTime=inf
  If : If  IfExpression=u1
  If1 : If  NumInputs=2  IfExpression=u1  ElseIfExpressions=u2  ShowElse=off
  Merge : Merge
  Relational Operator : RelationalOperator  OutDataTypeStr=boolean
  Terminator : Terminator
  Towards Failed : Subsystem  TreatAsAtomicUnit=on
  Towards Passed : Subsystem  TreatAsAtomicUnit=on
  Update to Failed : Subsystem  TreatAsAtomicUnit=on
  Update to Passed : Subsystem  TreatAsAtomicUnit=on
  counter : Merge
  Structvar_out : Outport
  wires:
  Structvar/1 -> Bus Assignment/1, Bus Selector/1
  Status/1 -> If/1
  If/1 -> Towards Failed/Action
  If/2 -> Towards Passed/Action
  [PosStep] -> Towards Failed/1(PosStep)
  [NegStep] -> Towards Passed/1(NegStep)
  Towards Failed/1(Out1) -> counter/1
  Towards Passed/1(Out1) -> counter/2
  [Cnt] -> Towards Failed/2(Cnt)
  [Thd] -> Towards Failed/3(Thd)
  Constant/1 -> Towards Passed/3(Thd)
  counter/1 -> [Cnt_update], Compare To Zero/1, Relational Operator/1
  Relational Operator/1 -> If1/1
  If1/1 -> Update to Failed/Action
  If1/2 -> Update to Passed/Action
  Compare To Zero/1 -> If1/2
  Enumerated Constant1/1 -> Update to Passed/1(In1)
  Update to Failed/1(Out1) -> Merge/1
  Update to Passed/1(Out1) -> Merge/2
  Enumerated Constant/1 -> Update to Failed/1(In1)
  Bus Assignment/1 -> Structvar_out/1
  Merge/1 -> [Sts_update]
  Bus Selector/1 -> [Cnt]  "<Cntr>"
  Bus Selector/3 -> [Thd]  "<Thd>"
  Bus Selector/4 -> [NegStep]  "<NegStep>"
  Bus Selector/5 -> [PosStep]  "<PosStep>"
  [Cnt_update] -> Bus Assignment/2
  [Sts_update] -> Bus Assignment/3
  [Cnt] -> Towards Passed/2(Cnt)
  [Thd] -> Relational Operator/2
  Bus Selector/2 -> Terminator/1  "<Sts>"

== system SF015A_WhlImbRejctn/WhlImbRejctn/WhlImbRejctnPer2/Flt Recovery- WhlSpdCorr Diag/CopyRight2 ==

== system SF015A_WhlImbRejctn/WhlImbRejctn/WhlImbRejctnPer2/Flt Recovery- WhlSpdCorr Diag/ElapsedTime1 ==
  FltStsTrue : Inport
  CopyRight2 : Subsystem  Description=|  mask(Copyright Information){none=on}
      | Copyright info block.                                               
      |                                                                     
      | Place copyright information at the top of every subsystem in design.
      mask prompts: none "No parameters"
      mask help: Place copyright information at the top of every subsystem in design.
      mask Display:
      | NxtrConf = 'Nexteer Confidential';
      | 
      | sys = bdroot; %handle for the current model ("system")
      | first = get_param(sys,'Created');
      | first = first(end-3:end);  %year is last four digits
      | 
      | last = get_param(sys,'LastModifiedDate');
      | if isempty(last)
      |     last = datestr(now,'yyyy');
      | else
      |     last = last(end-3:end);
      | end
      | 
      | if strcmp(first,last)
      |     fprintf('%s -- Copyright %s Nexteer',NxtrConf,first)
      | else
      |     fprintf('%s -- %s%s- %s Nexteer',NxtrConf,char(169),first,last)
      | end
  Data Store Read : DataStoreRead  Priority=1  DataStoreName=WhlSpdCorrlnDiagcLrngEnaPrev
      settings: AttributesFormatString="priority:  %<Priority>"
  Data Store Write : DataStoreWrite  Priority=2  DataStoreName=WhlSpdCorrlnDiagcLrngEnaPrev
      settings: AttributesFormatString="priority:  %<Priority>"
  If : If  NumInputs=2  IfExpression=u1  ElseIfExpressions=u2
  If not true elapsed time = 0 : Subsystem  TreatAsAtomicUnit=on
  "If true and last step is true calculate elapsed time " : Subsystem  TreatAsAtomicUnit=on
  "If true and last step not true elapsed time = 0 get reference time " : Subsystem  TreatAsAtomicUnit=on
  Logical Operator1 : Logic  Operator=NOT  AllPortsSameDT=off  OutDataTypeStr=boolean
  Logical Operator2 : Logic  Operator=NOT  AllPortsSameDT=off  OutDataTypeStr=boolean
  Merge : Merge  Inputs=3
  ElapsedTime : Outport
  wires:
  If/1 -> If not true elapsed time = 0/Action
  If/2 -> "If true and last step not true elapsed time = 0 get reference time "/Action
  If/3 -> "If true and last step is true calculate elapsed time "/Action
  If not true elapsed time = 0/1(SpanTi) -> Merge/1
  "If true and last step not true elapsed time = 0 get reference time "/1("SpanTi ") -> Merge/2
  "If true and last step is true calculate elapsed time "/1(SpanTi) -> Merge/3
  Merge/1 -> ElapsedTime/1
  FltStsTrue/1 -> Logical Operator2/1, Data Store Write/1
  Data Store Read/1 -> Logical Operator1/1
  Logical Operator2/1 -> If/1
  Logical Operator1/1 -> If/2

== system SF015A_WhlImbRejctn/WhlImbRejctn/WhlImbRejctnPer2/Flt Recovery- WhlSpdCorr Diag/FaultReset_Rcvry_False ==
  Action Port : ActionPort  ActionType=else
  Constant1 : Constant  Value=0  OutDataTypeStr=boolean
  CopyRight2 : Subsystem  Description=|  mask(Copyright Information){none=on}
      | Copyright info block.                                               
      |                                                                     
      | Place copyright information at the top of every subsystem in design.
      mask prompts: none "No parameters"
      mask help: Place copyright information at the top of every subsystem in design.
      mask Display:
      | NxtrConf = 'Nexteer Confidential';
      | 
      | sys = bdroot; %handle for the current model ("system")
      | first = get_param(sys,'Created');
      | first = first(end-3:end);  %year is last four digits
      | 
      | last = get_param(sys,'LastModifiedDate');
      | if isempty(last)
      |     last = datestr(now,'yyyy');
      | else
      |     last = last(end-3:end);
      | end
      | 
      | if strcmp(first,last)
      |     fprintf('%s -- Copyright %s Nexteer',NxtrConf,first)
      | else
      |     fprintf('%s -- %s%s- %s Nexteer',NxtrConf,char(169),first,last)
      | end
  Out1 : Outport
  wires:
  Constant1/1 -> Out1/1

== system SF015A_WhlImbRejctn/WhlImbRejctn/WhlImbRejctnPer2/Flt Recovery- WhlSpdCorr Diag/FaultReset_Rcvry_True ==
  Action Port : ActionPort  ActionType=then
  Constant15 : Constant  OutDataTypeStr=boolean
  CopyRight2 : Subsystem  Description=|  mask(Copyright Information){none=on}
      | Copyright info block.                                               
      |                                                                     
      | Place copyright information at the top of every subsystem in design.
      mask prompts: none "No parameters"
      mask help: Place copyright information at the top of every subsystem in design.
      mask Display:
      | NxtrConf = 'Nexteer Confidential';
      | 
      | sys = bdroot; %handle for the current model ("system")
      | first = get_param(sys,'Created');
      | first = first(end-3:end);  %year is last four digits
      | 
      | last = get_param(sys,'LastModifiedDate');
      | if isempty(last)
      |     last = datestr(now,'yyyy');
      | else
      |     last = last(end-3:end);
      | end
      | 
      | if strcmp(first,last)
      |     fprintf('%s -- Copyright %s Nexteer',NxtrConf,first)
      | else
      |     fprintf('%s -- %s%s- %s Nexteer',NxtrConf,char(169),first,last)
      | end
  Out1 : Outport
  wires:
  Constant15/1 -> Out1/1
